simulink model "building_HVAC_V00_027_AI_2019b"  (R2021b)
settings: Solver=ode3  StartTime=1425600  StopTime=1429297  FixedStep=0.1  RelTol=1e-3
model workspace (MAT data in the model file):
  A = 0
  pystep = 1
values from neighbouring files (symbols this model uses):
  Air_Cp = [1007 1007 1006 1006 1006 1006 1006 1006 1006 1006 1007 1007 ... (21 elements, 21x1)]    [data_07.mat]    (also in data_08.mat)
  Air_density = [1.783 1.582 1.422 1.367 1.341 1.316 1.292 1.268 1.246 1.225 1.204 1.184 ... (32 elements, 32x1)]    [data_07.mat]    (also in data_08.mat)
  Air_dynamic_viscosity_PaS = [1.318e-05 1.456e-05 1.588e-05 1.64e-05 1.665e-05 1.69e-05 1.715e-05 1.74e-05 1.764e-05 1.789e-05 1.813e-05 1.837e-05 ... (32 elements, 32x1)]    [data_07.mat]    (also in data_08.mat)
  Air_enthalpy = [325420 335490 345550 355620 365680 375730 385790 395850 405910 415970 426040 436110 ... (21 elements, 21x1)]    [data_07.mat]    (also in data_08.mat)
  Air_prandtl_number = [0.734 0.72 0.711 0.707 0.705 0.701 0.699 0.698 0.699 0.702]    [data_07.mat]    (also in data_08.mat)
  Air_Temp_for_Cp = [200 210 220 230 240 250 260 270 280 290 300 310 ... (21 elements, 21x1)]    [data_07.mat]    (also in data_08.mat)
  Air_Temp_for_density = [-75 -50 -25 -15 -10 -5 0 5 10 15 20 25 ... (32 elements, 32x1)]    [data_07.mat]    (also in data_08.mat)
  Air_Temp_for_dynamic_viscosity = [-75 -50 -25 -15 -10 -5 0 5 10 15 20 25 ... (32 elements, 32x1)]    [data_07.mat]    (also in data_08.mat)
  Air_Temp_for_enthalpy = [200 210 220 230 240 250 260 270 280 290 300 310 ... (21 elements, 21x1)]    [data_07.mat]    (also in data_08.mat)
  Air_Temp_for_prandtl_number = [-100 -50 0 25 50 100 150 200 250 300]    [data_07.mat]    (also in data_08.mat)
  Air_Temp_for_thermal_conductivity = [-190 -150 -100 -75 -50 -25 -15 -10 -5 0 5 10 ... (35 elements, 35x1)]    [data_07.mat]    (also in data_08.mat)
  Air_thermal_conductivity = [0.00782 0.01169 0.0162 0.01834 0.02041 0.02241 0.0232 0.02359 0.02397 0.02436 0.02474 0.02512 ... (35 elements, 35x1)]    [data_07.mat]    (also in data_08.mat)
  Ambient_Solar_heat_Seoul_20200701_to_20200731 = [0 0 0 0 0 0 2.777777778 38.88888889 72.22222222 97.22222222 333.3333333 263.8888889 ... (745 elements, 745x1)]    [data_07.mat]    (also in data_08.mat)
  Ambient_Solar_heat_Seoul_20200701_to_20210630 = [0 0 0 0 0 2.777777778 38.88888889 72.22222222 97.22222222 333.3333333 263.8888889 152.7777778 ... (8736 elements, 8736x1)]    [data_07.mat]    (also in data_08.mat)
  Ambient_Solar_heat_Seoul_20200801_to_20200831 = [0 0 0 0 0 0 2.777777778 11.11111111 38.88888889 63.88888889 127.7777778 258.3333333 ... (745 elements, 745x1)]    [data_07.mat]    (also in data_08.mat)
  Ambient_Solar_heat_Seoul_20200901_to_20200930 = [0 0 0 0 0 0 0 22.22222222 108.3333333 141.6666667 211.1111111 386.1111111 ... (721 elements, 721x1)]    [data_07.mat]    (also in data_08.mat)
  Ambient_Temp_Seoul_20200701_to_20200731 = [18.8 18.8 18.7 18.4 18.2 18.2 18.3 18.5 19.1 19.6 21.2 21.6 ... (745 elements, 745x1)]    [data_07.mat]    (also in data_08.mat)
  Ambient_Temp_Seoul_20200701_to_20210630 = [18.8 18.7 18.4 18.2 18.2 18.3 18.5 19.1 19.6 21.2 21.6 21.7 ... (8736 elements, 8736x1)]    [data_07.mat]    (also in data_08.mat)
  Ambient_Temp_Seoul_20200801_to_20200831 = [25 24.6 24.6 24.7 24.7 24.5 24.3 24.3 24.6 25 25.7 26.8 ... (745 elements, 745x1)]    [data_07.mat]    (also in data_08.mat)
  Ambient_Temp_Seoul_20200901_to_20200930 = [26.2 25.8 25.5 24.9 24.5 24.3 24 23.9 24.4 24.8 25.7 26.6 ... (721 elements, 721x1)]    [data_07.mat]    (also in data_08.mat)
  Ambient_Time_Seoul_20200701_to_20200731 = [0 3600 7200 10800 14400 18000 21600 25200 28800 32400 36000 39600 ... (745 elements, 745x1)]    [data_07.mat]    (also in data_08.mat)
  Ambient_Time_Seoul_20200701_to_20210630 = [0 3600 7200 10800 14400 18000 21600 25200 28800 32400 36000 39600 ... (8736 elements, 8736x1)]    [data_07.mat]    (also in data_08.mat)
  Ambient_Time_Seoul_20200901_to_20200930 = [0 3600 7200 10800 14400 18000 21600 25200 28800 32400 36000 39600 ... (721 elements, 721x1)]    [data_07.mat]    (also in data_08.mat)
  Ambient_Water_Vapor_Pressure_Seoul_20200701_to_20200731 = [18.4 18.8 18.6 18.2 17.9 17.7 18.6 18.6 18.5 19.1 19.9 19.5 ... (745 elements, 745x1)]    [data_07.mat]    (also in data_08.mat)
  Ambient_Water_Vapor_Pressure_Seoul_20200701_to_20210630 = [18.8 18.6 18.2 17.9 17.7 18.6 18.6 18.5 19.1 19.9 19.5 19.4 ... (8736 elements, 8736x1)]    [data_07.mat]    (also in data_08.mat)
  Ambient_Water_Vapor_Pressure_Seoul_20200801_to_20200831 = [28.4 27.7 28.1 28.8 29.1 28.8 28.8 29.1 29.7 30 31.3 29.8 ... (745 elements, 745x1)]    [data_07.mat]    (also in data_08.mat)
  Ambient_Water_Vapor_Pressure_Seoul_20200901_to_20200930 = [26.1 25.8 25.6 24.7 24 24.3 22.9 23.1 23.1 22.8 24 24.3 ... (721 elements, 721x1)]    [data_07.mat]    (also in data_08.mat)
  Ambient_wind_speed_Seoul_20200701_to_20200731 = [3.7 3 3 2.3 1.2 1.5 3.1 1.4 1 1.4 2.5 2.1 ... (745 elements, 745x1)]    [data_07.mat]    (also in data_08.mat)
  Ambient_wind_speed_Seoul_20200701_to_20210630 = [3 3 2.3 1.2 1.5 3.1 1.4 1 1.4 2.5 2.1 2 ... (8736 elements, 8736x1)]    [data_07.mat]    (also in data_08.mat)
  Ambient_wind_speed_Seoul_20200801_to_20200831 = [3.4 0.5 0.5 1.2 0.8 1.3 1.8 1.4 1.2 1.1 1.8 3.4 ... (745 elements, 745x1)]    [data_07.mat]    (also in data_08.mat)
  Ambient_wind_speed_Seoul_20200901_to_20200930 = [2.3 2.2 2.5 2.6 2.4 2.1 1.7 2.7 2.6 2.5 1.5 1.8 ... (721 elements, 721x1)]    [data_07.mat]    (also in data_08.mat)
  init_time = start_time +60    [SIMULINK_RUn.m]    (also in data_07.mat = 0; data_08.mat = 1425660)
  Initial_Temp = 273 + 28    (= 301)    [SIMULINK_RUn.m]    (also in data_07.mat = 285; data_08.mat = 302)
  Shadow_20200701_to_20210630 = [285 300 315 330 345 360 15 30 45 60 75 90 ... (8736 elements, 8736x1)]    [data_07.mat]    (also in data_08.mat)
  start_time = 12 * 3600 + da * day_to_sec    [SIMULINK_RUn.m]    (also in data_07.mat = 0; data_08.mat = 1425600)
  Under_30cm_ground_Temp_Seoul_20200701_to_20200731 = [22.6 22.6 22.5 22.5 22.4 22.3 22.3 22.2 22.1 22.1 22 22 ... (745 elements, 745x1)]    [data_07.mat]    (also in data_08.mat)
  Under_30cm_ground_Temp_Seoul_20200701_to_20210630 = [22.6 22.5 22.5 22.4 22.3 22.3 22.2 22.1 22.1 22 22 22 ... (8736 elements, 8736x1)]    [data_07.mat]    (also in data_08.mat)
  Under_30cm_ground_Temp_Seoul_20200801_to_20200831 = [25.6 25.6 25.6 25.5 25.5 25.5 25.4 25.4 25.3 25.3 25.3 25.2 ... (745 elements, 745x1)]    [data_07.mat]    (also in data_08.mat)
  Under_30cm_ground_Temp_Seoul_20200901_to_20200930 = [27.4 27.4 27.4 27.4 27.3 27.3 27.3 27.2 27.2 27.1 27 27 ... (721 elements, 721x1)]    [data_07.mat]    (also in data_08.mat)
  water_saturation_enthalpy_latent = [2500899.39 2498955.8 2496540.3 2494128 2491818 2489411 2487006 2484604 2482303 2479905 2477508 2475213 ... (64 elements, 64x1)]    [data_07.mat]    (also in data_08.mat)
  water_saturation_enthalpy_vapor = [2500900 2502500 2504300 2506100 2508000 2509800 2511600 2513400 2515300 2517100 2518900 2520800 ... (64 elements, 64x1)]    [data_07.mat]    (also in data_08.mat)
  water_saturation_pressure = [611.65 650.03 698.46 750.07 805.02 863.5 925.7 991.83 1062.2 1136.8 1216 1300 ... (64 elements, 64x1)]    [data_07.mat]    (also in data_08.mat)
  water_Temp_for_saturation_enthalpy_latent = [273.16 274 275 276 277 278 279 280 281 282 283 284 ... (64 elements, 64x1)]    [data_07.mat]    (also in data_08.mat)
  water_Temp_for_saturation_enthalpy_vapor = [273.16 274 275 276 277 278 279 280 281 282 283 284 ... (64 elements, 64x1)]    [data_07.mat]    (also in data_08.mat)
  water_Temp_for_saturation_pressure = [273.16 274 275 276 277 278 279 280 281 282 283 284 ... (64 elements, 64x1)]    [data_07.mat]    (also in data_08.mat)
undefined symbols (not defined in the file or in its folder): DiscIntNeverNeededParam
libraries: fuzblock x1
(part 2 of 3)

== system building_HVAC_V00_027_AI_2019b/Building_Block/Blower_and_InnerAir_Block ==
  Infiltration_[m3/s] : Inport
  Ventilation_[m3/s] : Inport  Port=2
  Ambient_temperature_[K]1 : Inport  Port=3
  Ambient_water_vapor_pressure_[Pa] : Inport  Port=4
  Blower_volume_flow_rate_[m3/s] : Inport  Port=5
  Q_AC_cooling_[W] : Inport  Port=6
  AC_ON : Inport  Port=7
  AC_Condensation_Mass_Flow_Rate_[kg/s]_Block : Subsystem
  AC_Outlet_Q_[W]_Block : Subsystem
  Absolute_Humidity_[-]_Block : Subsystem
  Air_Mass_Flow_Rate Infiltration InnerAir : Subsystem
  Air_Mass_Flow_Rate Ventilation InnerAir : Subsystem
  Blower_Mass_Flow_Rate_[kg/s] Water_and_Air : Subsystem
  Blower_Q_[W]_Block : Subsystem
  InnerAir_DewPoint_Temperature_[K]_Block : Subsystem
  InnerAir_H2O_Pressure_[Pa]_Block : Subsystem
  InnerAir_Temperature_Block : Subsystem
  Mass_H2O_vapor_InnerAir : Subsystem
  Mass_dry_air_InnerAir : Subsystem
  Water_Mass_Flow_Rate Infiltration InnerAir : Subsystem
  Water_Mass_Flow_Rate Ventilation InnerAir : Subsystem
  atmosperic pressure [Pa] : Constant  Value=101325
  gas constant dry air [J/kgK] : Constant  Value=287.05
  gas constant water [J/kgK] : Constant  Value=462.52
  InnerAir_temperature_[K] : Outport
  InnerAir_temperature_[degC] : Outport  Port=2
  tag scope: atmosphere_pressure=global, gas_constant_dry_air=global, gas_constant_water=global
  wires:
  atmosperic pressure [Pa]/1 -> [atmosphere_pressure]
  gas constant dry air [J/kgK]/1 -> [gas_constant_dry_air]
  gas constant water [J/kgK]/1 -> [gas_constant_water]
  Ventilation_[m3/s]/1 -> Water_Mass_Flow_Rate Ventilation InnerAir/1(Ventilation_[m3/s]), Air_Mass_Flow_Rate Ventilation InnerAir/1(Ventilation_[m3/s])
  Infiltration_[m3/s]/1 -> Water_Mass_Flow_Rate Infiltration InnerAir/3(Infiltration_[m3/s]), Air_Mass_Flow_Rate Infiltration InnerAir/1(Infiltration_[m3/s])
  Ambient_water_vapor_pressure_[Pa]/1 -> Water_Mass_Flow_Rate Infiltration InnerAir/1(Ambient_water_vapor_pressure_[Pa])
  Ambient_temperature_[K]1/1 -> Water_Mass_Flow_Rate Infiltration InnerAir/2(Ambient_temperature_[K]), Air_Mass_Flow_Rate Infiltration InnerAir/2(Ambient_temperature_[K]), Mass_H2O_vapor_InnerAir/1(Ambient_temperature_[K]2), Mass_dry_air_InnerAir/1(Ambient_temperature_[K]2)
  InnerAir_Temperature_Block/2(InnerAir_temperature_[degC]) -> InnerAir_temperature_[degC]/1
  Q_AC_cooling_[W]/1 -> AC_Condensation_Mass_Flow_Rate_[kg/s]_Block/1(Q_AC_cooling_[W])
  AC_ON/1 -> AC_Condensation_Mass_Flow_Rate_[kg/s]_Block/2(AC_ON)
  Blower_volume_flow_rate_[m3/s]/1 -> Blower_Mass_Flow_Rate_[kg/s] Water_and_Air/2(Blower_volume_flow_rate_[m3/s])
  InnerAir_Temperature_Block/1(InnerAir_temperature_[K]) -> InnerAir_temperature_[K]/1, Water_Mass_Flow_Rate Ventilation InnerAir/2(Inner_air_temperature_[K]), Air_Mass_Flow_Rate Ventilation InnerAir/2(InnerAir_temperature_[K]), Blower_Q_[W]_Block/1(Inner_air_temperature_[K]2), Blower_Mass_Flow_Rate_[kg/s] Water_and_Air/1(Inner_air_temperature_[K]1)

== system building_HVAC_V00_027_AI_2019b/Building_Block/East_Wall_Block ==
  Ambient_temperature_[K] : Inport
  Inner_air_temperature_[K] : Inport  Port=2
  Subsystem1 : Subsystem
  Subsystem2 : Subsystem
  Subsystem3 : Subsystem
  Subsystem4 : Subsystem
  East_outer_concrete_wall_temperature_[degC] : Outport
  East_insulator_temperature_[degC] : Outport  Port=2
  East_inner_concrete_wall_temperature_[degC] : Outport  Port=3
  Q_East_InnerWall_to_InnerAir_[W] : Outport  Port=4
  wires:
  Subsystem3/2(East_inner_concrete_wall_temperature_[degC]) -> East_inner_concrete_wall_temperature_[degC]/1
  Inner_air_temperature_[K]/1 -> Subsystem1/2(Inner_air_temperature_[K]), Subsystem3/2(Inner_air_temperature_[K])
  Subsystem4/2(East_insulator_temperature_[degC]) -> East_insulator_temperature_[degC]/1
  Subsystem1/1(Q_East_InnerWall_to_InnerAir_[W]) -> Q_East_InnerWall_to_InnerAir_[W]/1
  [Inside] -> Subsystem3/3(East_Inner_Convective_coefficient_h), Subsystem1/3(East_Inner_Convective_coefficient_h)
  Subsystem2/1(East_outer_concrete_wall_temperature_[K]) -> Subsystem4/1(East_Outer_concrete_wall_temperature_[K])
  Subsystem4/1(East_insulator_temperature_[K]) -> Subsystem3/1(East_Insulator_temperature_[K]), Subsystem2/2(East_Insulator_temperature_[K])
  Ambient_temperature_[K]/1 -> Subsystem2/1(Ambient_temperature_[K])
  [Outside_East_West] -> Subsystem2/3(East_Out_Convective_coefficient_h)
  Subsystem2/2(East_outer_concrete_wall_temperature_[degC]) -> East_outer_concrete_wall_temperature_[degC]/1
  Subsystem3/1(East_inner_concrete_wall_temperature_[K]) -> Subsystem1/1(East_inner_concrete_wall_temperature_[K]), Subsystem4/2(East_Inner_concrete_wall_temperature_[K])

== system building_HVAC_V00_027_AI_2019b/Building_Block/Floorl_Block ==
  Under_30cm_soil_temperature_[K] : Inport
  Inner_air_temperature_[K] : Inport  Port=2
  Subsystem1 : Subsystem
  Subsystem3 : Subsystem
  Subsystem4 : Subsystem
  Floor_insulator_temperature_[degC] : Outport
  Floor_inner_wall_temperature_[degC] : Outport  Port=2
  Q_floor_to_InnerAir_[W] : Outport  Port=3
  wires:
  Subsystem3/1(Floor_inner_wall_temperature_[K]) -> Subsystem1/1(Floor_inner_concrete_wall_temperature_[K]), Subsystem4/2(Floor_Inner_concrete_wall_temperature_[K])
  Under_30cm_soil_temperature_[K]/1 -> Subsystem4/1(Under_30cm_soil_temperature_[K])
  Subsystem4/1(Floor_insulator_temperature_[K]) -> Subsystem3/1(Floor_Insulator_temperature_[K])
  [Inside] -> Subsystem1/3(West_Inner_Convective_coefficient_h), Subsystem3/3(Floor_Inner_Convective_coefficient_h)
  Subsystem1/1(Q_Floor_InnerWall_to_InnerAir_[W]) -> Q_floor_to_InnerAir_[W]/1
  Subsystem4/2(Floor_insulator_temperature_[degC]) -> Floor_insulator_temperature_[degC]/1
  Inner_air_temperature_[K]/1 -> Subsystem1/2(Inner_air_temperature_[K]), Subsystem3/2(Inner_air_temperature_[K])
  Subsystem3/2(Floor_inner_wall_temperature_[degC]) -> Floor_inner_wall_temperature_[degC]/1

== system building_HVAC_V00_027_AI_2019b/Building_Block/North_Wall_Block ==
  Ambient_temperature_[K] : Inport
  Inner_air_temperature_[K] : Inport  Port=2
  Subsystem1 : Subsystem
  Subsystem2 : Subsystem
  Subsystem3 : Subsystem
  Subsystem4 : Subsystem
  North_outer_concrete_wall_temperature_[degC] : Outport
  North_insulator_temperature_[degC] : Outport  Port=2
  North_inner_concrete_wall_temperature_[degC] : Outport  Port=3
  Q_North_InnerWall_to_InnerAir_[W] : Outport  Port=4
  wires:
  Subsystem3/2(North_inner_concrete_wall_temperature_[degC]) -> North_inner_concrete_wall_temperature_[degC]/1
  Inner_air_temperature_[K]/1 -> Subsystem1/2(Inner_air_temperature_[K]), Subsystem3/2(Inner_air_temperature_[K])
  Subsystem4/2(North_insulator_temperature_[degC]) -> North_insulator_temperature_[degC]/1
  Subsystem1/1(Q_North_InnerWall_to_InnerAir_[W]) -> Q_North_InnerWall_to_InnerAir_[W]/1
  [Inside] -> Subsystem3/3(North_Inner_Convective_coefficient_h), Subsystem1/3(North_Inner_Convective_coefficient_h)
  Subsystem2/1(North_outer_concrete_wall_temperature_[K]) -> Subsystem4/1(North_Outer_concrete_wall_temperature_[K])
  Subsystem4/1(North_insulator_temperature_[K]) -> Subsystem3/1(North_Insulator_temperature_[K]), Subsystem2/2(North_Insulator_temperature_[K])
  Ambient_temperature_[K]/1 -> Subsystem2/1(Ambient_temperature_[K])
  [Outside_South_North] -> Subsystem2/3(North_Out_Convective_coefficient_h)
  Subsystem2/2(North_outer_concrete_wall_temperature_[degC]) -> North_outer_concrete_wall_temperature_[degC]/1
  Subsystem3/1(North_inner_concrete_wall_temperature_[K]) -> Subsystem1/1(North_inner_concrete_wall_temperature_[K]), Subsystem4/2(North_Inner_concrete_wall_temperature_[K])

== system building_HVAC_V00_027_AI_2019b/Building_Block/South_Wall_Block ==
  Ambient_temperature_[K] : Inport
  Inner_air_temperature_[K] : Inport  Port=2
  Subsystem1 : Subsystem
  Subsystem2 : Subsystem
  Subsystem3 : Subsystem
  Subsystem4 : Subsystem
  South_outer_concrete_wall_temperature_[degC] : Outport
  South_insulator_temperature_[degC] : Outport  Port=2
  South_inner_concrete_wall_temperature_[degC] : Outport  Port=3
  Q_South_InnerWall_to_InnerAir_[W] : Outport  Port=4
  wires:
  Subsystem3/1(South_inner_concrete_wall_temperature_[K]) -> Subsystem1/1(South_inner_concrete_wall_temperature_[K]), Subsystem4/2(South_Inner_concrete_wall_temperature_[K])
  Subsystem2/2(South_outer_concrete_wall_temperature_[degC]) -> South_outer_concrete_wall_temperature_[degC]/1
  [Outside_South_North] -> Subsystem2/3(South_Out_Convective_coefficient_h)
  Ambient_temperature_[K]/1 -> Subsystem2/1(Ambient_temperature_[K])
  Subsystem4/1(South_insulator_temperature_[K]) -> Subsystem2/2(South_Insulator_temperature_[K]), Subsystem3/1(South_Insulator_temperature_[K])
  Subsystem2/1(South_outer_concrete_wall_temperature_[K]) -> Subsystem4/1(South_Outer_concrete_wall_temperature_[K])
  [Inside] -> Subsystem3/3(South_Inner_Convective_coefficient_h), Subsystem1/3(South_Inner_Convective_coefficient_h)
  Subsystem1/1(Q_South_InnerWall_to_InnerAir_[W]) -> Q_South_InnerWall_to_InnerAir_[W]/1
  Subsystem4/2(South_insulator_temperature_[degC]) -> South_insulator_temperature_[degC]/1
  Inner_air_temperature_[K]/1 -> Subsystem3/2(Inner_air_temperature_[K]), Subsystem1/2(Inner_air_temperature_[K])
  Subsystem3/2(South_inner_concrete_wall_temperature_[degC]) -> South_inner_concrete_wall_temperature_[degC]/1

== system building_HVAC_V00_027_AI_2019b/Building_Block/Subsystem ==
  Density : Inport
  Wind speed (m/s) : Inport  Port=2
  Dynamic viscosity : Inport  Port=3
  Ptandtl number : Inport  Port=4
  Air Thermal conductivity(W/mK) : Inport  Port=5
  Characteristic_length_(m) L : Inport  Port=6
  "Convective_coefficient_(W/(m2)K) h=(Nu)x(k)/(L) Frank P. Incropera and David P. DeWitt, \"Fundamentals of Heat and Mass Transfer\", (1996), FOURTH EDITION, pg. 320" : Fcn  Expr=u(1)/u(2)*u(3)
  Mux1 : Mux
  Mux2 : Mux  Inputs=2
  Mux3 : Mux  Inputs=3
  "Nusselt_number_(-) Nu [laminar_flow] Frank P. Incropera and David P. DeWitt, \"Fundamentals of Heat and Mass Transfer\", (1996), FOURTH EDITION, pg. 354" : Fcn  Expr=0.664*(u(1)^(1/2))*(u(2)^(1/3))
  "Nusselt_number_(-) Nu [turbulent_flow] Frank P. Incropera and David P. DeWitt, \"Fundamentals of Heat and Mass Transfer\", (1996), FOURTH EDITION, pg. 355" : Fcn  Expr=0.0296*(u(1)^(4/5))*(u(2)^(1/3))
  Reynold_number_(-) Re : Fcn  Expr=u(1)*u(2)*u(3)/u(4)
  Switch1 : Switch  Criteria=u2 > Threshold  Threshold=10^8
  h (W/(m2)K) : Outport  VectorParamsAs1DForOutWhenUnconnected=off
  wires:
  Mux2/1 -> "Nusselt_number_(-) Nu [turbulent_flow] Frank P. Incropera and David P. DeWitt, \"Fundamentals of Heat and Mass Transfer\", (1996), FOURTH EDITION, pg. 355"/1, "Nusselt_number_(-) Nu [laminar_flow] Frank P. Incropera and David P. DeWitt, \"Fundamentals of Heat and Mass Transfer\", (1996), FOURTH EDITION, pg. 354"/1
  "Nusselt_number_(-) Nu [laminar_flow] Frank P. Incropera and David P. DeWitt, \"Fundamentals of Heat and Mass Transfer\", (1996), FOURTH EDITION, pg. 354"/1 -> Switch1/3
  "Nusselt_number_(-) Nu [turbulent_flow] Frank P. Incropera and David P. DeWitt, \"Fundamentals of Heat and Mass Transfer\", (1996), FOURTH EDITION, pg. 355"/1 -> Switch1/1
  Mux1/1 -> Reynold_number_(-) Re/1
  Characteristic_length_(m) L/1 -> Mux3/2, Mux1/3
  Mux3/1 -> "Convective_coefficient_(W/(m2)K) h=(Nu)x(k)/(L) Frank P. Incropera and David P. DeWitt, \"Fundamentals of Heat and Mass Transfer\", (1996), FOURTH EDITION, pg. 320"/1
  Ptandtl number/1 -> Mux2/2
  Switch1/1 -> Mux3/1
  Reynold_number_(-) Re/1 -> Switch1/2, Mux2/1
  Dynamic viscosity/1 -> Mux1/4
  Air Thermal conductivity(W/mK)/1 -> Mux3/3
  Density/1 -> Mux1/1
  "Convective_coefficient_(W/(m2)K) h=(Nu)x(k)/(L) Frank P. Incropera and David P. DeWitt, \"Fundamentals of Heat and Mass Transfer\", (1996), FOURTH EDITION, pg. 320"/1 -> h (W/(m2)K)/1
  Wind speed (m/s)/1 -> Mux1/2

== system building_HVAC_V00_027_AI_2019b/Building_Block/Subsystem1 ==
  Density : Inport
  Wind speed (m/s) : Inport  Port=2
  Dynamic viscosity : Inport  Port=3
  Ptandtl number : Inport  Port=4
  Air Thermal conductivity(W/mK) : Inport  Port=5
  Characteristic_length_(m) L : Inport  Port=6
  "Convective_coefficient_(W/(m2)K) h=(Nu)x(k)/(L) Frank P. Incropera and David P. DeWitt, \"Fundamentals of Heat and Mass Transfer\", (1996), FOURTH EDITION, pg. 320" : Fcn  Expr=u(1)/u(2)*u(3)
  Mux1 : Mux
  Mux2 : Mux  Inputs=2
  Mux3 : Mux  Inputs=3
  "Nusselt_number_(-) Nu [laminar_flow] Frank P. Incropera and David P. DeWitt, \"Fundamentals of Heat and Mass Transfer\", (1996), FOURTH EDITION, pg. 354" : Fcn  Expr=0.664*(u(1)^(1/2))*(u(2)^(1/3))
  "Nusselt_number_(-) Nu [turbulent_flow] Frank P. Incropera and David P. DeWitt, \"Fundamentals of Heat and Mass Transfer\", (1996), FOURTH EDITION, pg. 355" : Fcn  Expr=0.0296*(u(1)^(4/5))*(u(2)^(1/3))
  Reynold_number_(-) Re : Fcn  Expr=u(1)*u(2)*u(3)/u(4)
  Switch1 : Switch  Criteria=u2 > Threshold  Threshold=10^8
  h (W/(m2)K) : Outport  VectorParamsAs1DForOutWhenUnconnected=off
  wires:
  Wind speed (m/s)/1 -> Mux1/2
  "Convective_coefficient_(W/(m2)K) h=(Nu)x(k)/(L) Frank P. Incropera and David P. DeWitt, \"Fundamentals of Heat and Mass Transfer\", (1996), FOURTH EDITION, pg. 320"/1 -> h (W/(m2)K)/1
  Density/1 -> Mux1/1
  Air Thermal conductivity(W/mK)/1 -> Mux3/3
  Dynamic viscosity/1 -> Mux1/4
  Reynold_number_(-) Re/1 -> Mux2/1, Switch1/2
  Switch1/1 -> Mux3/1
  Ptandtl number/1 -> Mux2/2
  Mux3/1 -> "Convective_coefficient_(W/(m2)K) h=(Nu)x(k)/(L) Frank P. Incropera and David P. DeWitt, \"Fundamentals of Heat and Mass Transfer\", (1996), FOURTH EDITION, pg. 320"/1
  Characteristic_length_(m) L/1 -> Mux1/3, Mux3/2
  Mux1/1 -> Reynold_number_(-) Re/1
  "Nusselt_number_(-) Nu [turbulent_flow] Frank P. Incropera and David P. DeWitt, \"Fundamentals of Heat and Mass Transfer\", (1996), FOURTH EDITION, pg. 355"/1 -> Switch1/1
  "Nusselt_number_(-) Nu [laminar_flow] Frank P. Incropera and David P. DeWitt, \"Fundamentals of Heat and Mass Transfer\", (1996), FOURTH EDITION, pg. 354"/1 -> Switch1/3
  Mux2/1 -> "Nusselt_number_(-) Nu [laminar_flow] Frank P. Incropera and David P. DeWitt, \"Fundamentals of Heat and Mass Transfer\", (1996), FOURTH EDITION, pg. 354"/1, "Nusselt_number_(-) Nu [turbulent_flow] Frank P. Incropera and David P. DeWitt, \"Fundamentals of Heat and Mass Transfer\", (1996), FOURTH EDITION, pg. 355"/1

== system building_HVAC_V00_027_AI_2019b/Building_Block/West_Wall_Block ==
  Ambient_temperature_[K] : Inport
  Inner_air_temperature_[K] : Inport  Port=2
  Subsystem1 : Subsystem
  Subsystem2 : Subsystem
  Subsystem3 : Subsystem
  Subsystem4 : Subsystem
  West_outer_concrete_wall_temperature_[degC] : Outport
  West_insulator_temperature_[degC] : Outport  Port=2
  West_inner_concrete_wall_temperature_[degC] : Outport  Port=3
  Q_West_InnerWall_to_InnerAir_[W] : Outport  Port=4
  wires:
  Subsystem3/1(West_inner_concrete_wall_temperature_[K]) -> Subsystem1/1(West_inner_concrete_wall_temperature_[K]), Subsystem4/2(West_Inner_concrete_wall_temperature_[K])
  Subsystem2/2(West_outer_concrete_wall_temperature_[degC]) -> West_outer_concrete_wall_temperature_[degC]/1
  [Outside_East_West] -> Subsystem2/3(West_Out_Convective_coefficient_h)
  Ambient_temperature_[K]/1 -> Subsystem2/1(Ambient_temperature_[K])
  Subsystem4/1(West_insulator_temperature_[K]) -> Subsystem2/2(West_Insulator_temperature_[K]), Subsystem3/1(West_Insulator_temperature_[K])
  Subsystem2/1(West_outer_concrete_wall_temperature_[K]) -> Subsystem4/1(West_Outer_concrete_wall_temperature_[K])
  [Inside] -> Subsystem1/3(West_Inner_Convective_coefficient_h), Subsystem3/3(West_Inner_Convective_coefficient_h)
  Subsystem1/1(Q_West_InnerWall_to_InnerAir_[W]) -> Q_West_InnerWall_to_InnerAir_[W]/1
  Subsystem4/2(West_insulator_temperature_[degC]) -> West_insulator_temperature_[degC]/1
  Inner_air_temperature_[K]/1 -> Subsystem1/2(Inner_air_temperature_[K]), Subsystem3/2(Inner_air_temperature_[K])
  Subsystem3/2(West_inner_concrete_wall_temperature_[degC]) -> West_inner_concrete_wall_temperature_[degC]/1

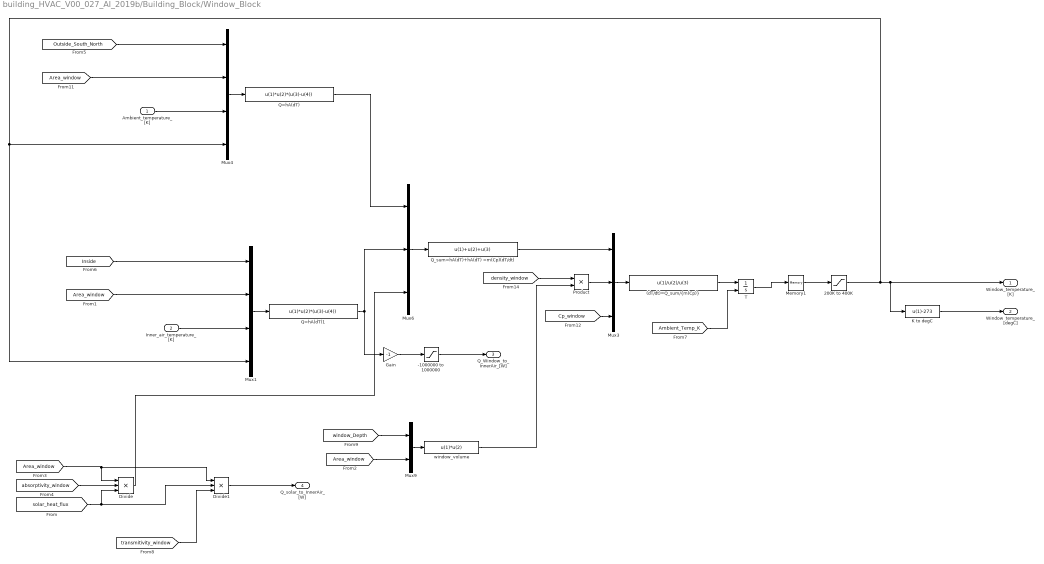
== system building_HVAC_V00_027_AI_2019b/Building_Block/Window_Block ==
  Ambient_temperature_[K] : Inport
  Inner_air_temperature_[K] : Inport  Port=2
  "(dT/dt)=Q_sum/{m(Cp)}" : Fcn  Expr=u(1)/u(2)/u(3)
  -1000000 to 1000000 : Saturate  UpperLimit=1000000  LowerLimit=-1000000
  200K to 400K : Saturate  UpperLimit=400  LowerLimit=200
  Divide : Product  Inputs=***
  Divide1 : Product  Inputs=***
  Gain : Gain  Gain=-1
  K to degC : Fcn  Expr=u(1)-273
  Memory1 : Memory  InitialCondition=300  InheritSampleTime=on
  Mux1 : Mux
  Mux3 : Mux  Inputs=3
  Mux4 : Mux
  Mux6 : Mux  Inputs=3
  Mux9 : Mux  Inputs=2
  Product : Product
  Q=hA(dT) : Fcn  Expr=u(1)*u(2)*(u(3)-u(4))
  Q=hA(dT)1 : Fcn  Expr=u(1)*u(2)*(u(3)-u(4))
  Q_sum=hA(dT)+hA(dT) =m(Cp)(dT/dt) : Fcn  Expr=u(1)+u(2)+u(3)
  T : Integrator  InitialConditionSource=external
  window_volume : Fcn  Expr=u(1)*u(2)
  Window_temperature_[K] : Outport
  Window_temperature_[degC] : Outport  Port=2
  Q_Window_to_InnerAir_[W] : Outport  Port=3
  Q_solar_to_InnerAir_[W] : Outport  Port=4
  wires:
  Mux6/1 -> Q_sum=hA(dT)+hA(dT) =m(Cp)(dT/dt)/1
  Mux3/1 -> "(dT/dt)=Q_sum/{m(Cp)}"/1
  [density_window] -> Product/1
  Mux9/1 -> window_volume/1
  "(dT/dt)=Q_sum/{m(Cp)}"/1 -> T/1
  [Cp_window] -> Mux3/3
  Product/1 -> Mux3/2
  [window_Depth] -> Mux9/1
  [Area_window] -> Mux9/2
  T/1 -> Memory1/1
  Q=hA(dT)1/1 -> Gain/1, Mux6/2
  Memory1/1 -> 200K to 400K/1
  Q=hA(dT)/1 -> Mux6/1
  Q_sum=hA(dT)+hA(dT) =m(Cp)(dT/dt)/1 -> Mux3/1
  window_volume/1 -> Product/2
  K to degC/1 -> Window_temperature_[degC]/1
  [Area_window] -> Mux4/2
  Ambient_temperature_[K]/1 -> Mux4/3
  Mux4/1 -> Q=hA(dT)/1
  [Outside_South_North] -> Mux4/1
  200K to 400K/1 -> Mux4/4, Mux1/4, K to degC/1, Window_temperature_[K]/1
  [Inside] -> Mux1/1
  Mux1/1 -> Q=hA(dT)1/1
  Inner_air_temperature_[K]/1 -> Mux1/3
  [Area_window] -> Mux1/2
  -1000000 to 1000000/1 -> Q_Window_to_InnerAir_[W]/1
  Gain/1 -> -1000000 to 1000000/1
  Divide/1 -> Mux6/3
  Divide1/1 -> Q_solar_to_InnerAir_[W]/1
  [Area_window] -> Divide1/1, Divide/1
  [solar_heat_flux] -> Divide1/2, Divide/3
  [absorptivity_window] -> Divide/2
  [Ambient_Temp_K] -> T/2
  [transmitivity_window] -> Divide1/3

== system building_HVAC_V00_027_AI_2019b/Building_Block/Blower_and_InnerAir_Block/AC_Condensation_Mass_Flow_Rate_[kg//s]_Block ==
  Q_AC_cooling_[W] : Inport
  AC_ON : Inport  Port=2
  Divide : Product  Inputs=**/
  Latent_enthalpy_of_saturated_water_(J/kg) of temperature_(K)1 : Lookup_n-D  NumberOfTableDimensions=1  BreakpointsForDimension1=water_Temp_for_saturation_enthalpy_latent  Table=water_saturation_enthalpy_latent  InternalRulePriority=Speed  RndMeth=Simplest  InputSameDT=on
  Saturation1 : Saturate  UpperLimit=100  LowerLimit=0
  Saturation5 : Saturate  UpperLimit=400  LowerLimit=273.16
  Scope25 : Scope
  "[J/kg]" : Gain
  "[K]1" : Gain
  "[W]" : Gain
  "[kg/s]1" : Gain
  tag scope: AC_condensation_mass_flow=global
  wires:
  Divide/1 -> Saturation1/1
  [dewpoint_temperature_H2O_vapor] -> "[K]1"/1
  "[J/kg]"/1 -> Divide/3
  "[K]1"/1 -> Saturation5/1
  "[kg/s]1"/1 -> Scope25/1, [AC_condensation_mass_flow]
  Saturation5/1 -> Latent_enthalpy_of_saturated_water_(J/kg) of temperature_(K)1/1
  Latent_enthalpy_of_saturated_water_(J/kg) of temperature_(K)1/1 -> "[J/kg]"/1
  Q_AC_cooling_[W]/1 -> "[W]"/1
  AC_ON/1 -> Divide/1
  "[W]"/1 -> Divide/2
  Saturation1/1 -> "[kg/s]1"/1

== system building_HVAC_V00_027_AI_2019b/Building_Block/Blower_and_InnerAir_Block/AC_Outlet_Q_[W]_Block ==
  Add1 : Sum
  Add2 : Sum  Inputs=+-
  Divide2 : Product  Inputs=**
  Divide3 : Product  Inputs=**
  Enthalpy_of_air_(J/kg) of temperature_(K)1 : Lookup_n-D  NumberOfTableDimensions=1  BreakpointsForDimension1=Air_Temp_for_enthalpy  Table=Air_enthalpy  InternalRulePriority=Speed  RndMeth=Simplest  InputSameDT=on
  Enthalpy_of_saturated_water_vapor_(J/kg) of temperature_(K)1 : Lookup_n-D  NumberOfTableDimensions=1  BreakpointsForDimension1=water_Temp_for_saturation_enthalpy_vapor  Table=water_saturation_enthalpy_vapor  InternalRulePriority=Speed  RndMeth=Simplest  InputSameDT=on
  Saturation3 : Saturate  UpperLimit=400  LowerLimit=273.16
  Saturation6 : Saturate  UpperLimit=400  LowerLimit=200
  Scope1 : Scope
  Scope2 : Scope
  Scope3 : Scope
  "[J/kg]2" : Gain
  "[J/kg]3" : Gain
  "[K]3" : Gain
  "[K]4" : Gain
  "[kg/s]3" : Gain
  "[kg/s]4" : Gain
  tag scope: AC_outlet_Q=global
  wires:
  [dewpoint_temperature_H2O_vapor] -> Scope3/1, "[K]4"/1, "[K]3"/1
  [Blower_mass_flow_rate_air] -> "[kg/s]4"/1
  Add2/1 -> Scope2/1, "[kg/s]3"/1
  "[J/kg]3"/1 -> Divide3/2
  Enthalpy_of_air_(J/kg) of temperature_(K)1/1 -> "[J/kg]3"/1
  Saturation6/1 -> Enthalpy_of_air_(J/kg) of temperature_(K)1/1
  Divide2/1 -> Add1/1
  "[K]4"/1 -> Saturation6/1
  "[J/kg]2"/1 -> Divide2/2
  Divide3/1 -> Add1/2
  Add1/1 -> [AC_outlet_Q], Scope1/1
  Enthalpy_of_saturated_water_vapor_(J/kg) of temperature_(K)1/1 -> "[J/kg]2"/1
  Saturation3/1 -> Enthalpy_of_saturated_water_vapor_(J/kg) of temperature_(K)1/1
  "[kg/s]3"/1 -> Divide2/1
  "[K]3"/1 -> Saturation3/1
  "[kg/s]4"/1 -> Divide3/1
  [Blower_mass_flow_rate_water] -> Add2/1
  [AC_condensation_mass_flow] -> Add2/2

== system building_HVAC_V00_027_AI_2019b/Building_Block/Blower_and_InnerAir_Block/Absolute_Humidity_[-]_Block ==
  M_H2O_vapor / M_dry_air : Fcn  Expr=u(1)/u(2)
  Mux1 : Mux  Inputs=2
  Saturation1 : Saturate  UpperLimit=1  LowerLimit=0
  tag scope: absolute_humidity=global
  wires:
  Mux1/1 -> M_H2O_vapor / M_dry_air/1
  [M_dry_air] -> Mux1/2
  M_H2O_vapor / M_dry_air/1 -> Saturation1/1
  [M_H20_vapor] -> Mux1/1
  Saturation1/1 -> [absolute_humidity]

== system building_HVAC_V00_027_AI_2019b/Building_Block/Blower_and_InnerAir_Block/Air_Mass_Flow_Rate Infiltration InnerAir ==
  Infiltration_[m3/s] : Inport
  Ambient_temperature_[K] : Inport  Port=2
  Mux8 : Mux
  m_dot = P(V_dot)/R/T : Fcn  Expr=u(1)*u(2)/u(3)/u(4)
  tag scope: Infiltration_air=global
  wires:
  [atmosphere_pressure] -> Mux8/1
  [gas_constant_dry_air] -> Mux8/3
  Mux8/1 -> m_dot = P(V_dot)/R/T/1
  m_dot = P(V_dot)/R/T/1 -> [Infiltration_air]
  Ambient_temperature_[K]/1 -> Mux8/4
  Infiltration_[m3/s]/1 -> Mux8/2

== system building_HVAC_V00_027_AI_2019b/Building_Block/Blower_and_InnerAir_Block/Air_Mass_Flow_Rate Ventilation InnerAir ==
  Ventilation_[m3/s] : Inport
  InnerAir_temperature_[K] : Inport  Port=2
  Mux9 : Mux
  m_dot = P(V_dot)/R/T1 : Fcn  Expr=u(1)*u(2)/u(3)/u(4)
  tag scope: Ventilation_air=global
  wires:
  m_dot = P(V_dot)/R/T1/1 -> [Ventilation_air]
  [gas_constant_dry_air] -> Mux9/3
  [pressure_H2O_vapor] -> Mux9/1
  Mux9/1 -> m_dot = P(V_dot)/R/T1/1
  Ventilation_[m3/s]/1 -> Mux9/2
  InnerAir_temperature_[K]/1 -> Mux9/4

== system building_HVAC_V00_027_AI_2019b/Building_Block/Blower_and_InnerAir_Block/Blower_Mass_Flow_Rate_[kg//s] Water_and_Air ==
  Inner_air_temperature_[K]1 : Inport
  Blower_volume_flow_rate_[m3/s] : Inport  Port=2
  Mux12 : Mux
  Mux13 : Mux
  Scope1 : Scope
  Scope24 : Scope
  m_dot = P(V_dot)/R/T4 : Fcn  Expr=u(1)*u(2)/u(3)/u(4)
  m_dot = P(V_dot)/R/T5 : Fcn  Expr=u(1)*u(2)/u(3)/u(4)
  tag scope: Blower_mass_flow_rate_air=global, Blower_mass_flow_rate_water=global
  wires:
  [gas_constant_dry_air] -> Mux12/3
  Inner_air_temperature_[K]1/1 -> Mux12/4, Mux13/4
  [atmosphere_pressure] -> Mux12/1
  Blower_volume_flow_rate_[m3/s]/1 -> Mux13/2, Mux12/2
  Mux12/1 -> m_dot = P(V_dot)/R/T4/1
  Mux13/1 -> m_dot = P(V_dot)/R/T5/1
  [gas_constant_water] -> Mux13/3
  [pressure_H2O_vapor] -> Mux13/1
  m_dot = P(V_dot)/R/T4/1 -> Scope24/1, [Blower_mass_flow_rate_air]
  m_dot = P(V_dot)/R/T5/1 -> Scope1/1, [Blower_mass_flow_rate_water]

== system building_HVAC_V00_027_AI_2019b/Building_Block/Blower_and_InnerAir_Block/Blower_Q_[W]_Block ==
  Inner_air_temperature_[K]2 : Inport
  Add1 : Sum
  Divide2 : Product  Inputs=**
  Divide3 : Product  Inputs=**
  Enthalpy_of_air_(J/kg) of temperature_(K)2 : Lookup_n-D  NumberOfTableDimensions=1  BreakpointsForDimension1=Air_Temp_for_enthalpy  Table=Air_enthalpy  InternalRulePriority=Speed  RndMeth=Simplest  InputSameDT=on
  Enthalpy_of_saturated_water_vapor_(J/kg) of temperature_(K)1 : Lookup_n-D  NumberOfTableDimensions=1  BreakpointsForDimension1=water_Temp_for_saturation_enthalpy_vapor  Table=water_saturation_enthalpy_vapor  InternalRulePriority=Speed  RndMeth=Simplest  InputSameDT=on
  Saturation3 : Saturate  UpperLimit=400  LowerLimit=273.16
  Saturation6 : Saturate  UpperLimit=400  LowerLimit=200
  Scope24 : Scope
  "[J/kg]2" : Gain
  "[J/kg]3" : Gain
  "[K]3" : Gain
  "[K]4" : Gain
  "[kg/s]3" : Gain
  "[kg/s]4" : Gain
  tag scope: Blower_Q=global
  wires:
  Saturation3/1 -> Enthalpy_of_saturated_water_vapor_(J/kg) of temperature_(K)1/1
  [Blower_mass_flow_rate_water] -> "[kg/s]3"/1
  "[K]3"/1 -> Saturation3/1
  "[J/kg]2"/1 -> Divide2/2
  Inner_air_temperature_[K]2/1 -> "[K]4"/1, "[K]3"/1
  "[kg/s]4"/1 -> Divide3/1
  "[kg/s]3"/1 -> Divide2/1
  Add1/1 -> Scope24/1, [Blower_Q]
  [Blower_mass_flow_rate_air] -> "[kg/s]4"/1
  Divide3/1 -> Add1/2
  Enthalpy_of_saturated_water_vapor_(J/kg) of temperature_(K)1/1 -> "[J/kg]2"/1
  "[K]4"/1 -> Saturation6/1
  "[J/kg]3"/1 -> Divide3/2
  Enthalpy_of_air_(J/kg) of temperature_(K)2/1 -> "[J/kg]3"/1
  Saturation6/1 -> Enthalpy_of_air_(J/kg) of temperature_(K)2/1
  Divide2/1 -> Add1/1

== system building_HVAC_V00_027_AI_2019b/Building_Block/Blower_and_InnerAir_Block/InnerAir_DewPoint_Temperature_[K]_Block ==
  DewPoint_temperature_[K] of H2O_pressure_[Pa] : Lookup_n-D  NumberOfTableDimensions=1  BreakpointsForDimension1=water_saturation_pressure  Table=water_Temp_for_saturation_pressure  InternalRulePriority=Speed  RndMeth=Simplest  InputSameDT=on
  Saturation7 : Saturate  UpperLimit=245779  LowerLimit=611.65
  tag scope: dewpoint_temperature_H2O_vapor=global
  wires:
  Saturation7/1 -> DewPoint_temperature_[K] of H2O_pressure_[Pa]/1
  DewPoint_temperature_[K] of H2O_pressure_[Pa]/1 -> [dewpoint_temperature_H2O_vapor]
  [pressure_H2O_vapor] -> Saturation7/1

== system building_HVAC_V00_027_AI_2019b/Building_Block/Blower_and_InnerAir_Block/InnerAir_H2O_Pressure_[Pa]_Block ==
  Mux2 : Mux  Inputs=2
  "P_H2O_vapor = (omega)(P)/{0.622+omega}" : Fcn  Expr=u(1)*u(2)/(0.622+u(1))
  tag scope: pressure_H2O_vapor=global
  wires:
  [atmosphere_pressure] -> Mux2/2
  Mux2/1 -> "P_H2O_vapor = (omega)(P)/{0.622+omega}"/1
  "P_H2O_vapor = (omega)(P)/{0.622+omega}"/1 -> [pressure_H2O_vapor]
  [absolute_humidity] -> Mux2/1

== system building_HVAC_V00_027_AI_2019b/Building_Block/Blower_and_InnerAir_Block/InnerAir_Temperature_Block ==
  Air_Cp_(J/kgK) of temperature_(K) : Lookup_n-D  NumberOfTableDimensions=1  BreakpointsForDimension1=Air_Temp_for_Cp  Table=Air_Cp  InternalRulePriority=Speed  RndMeth=Simplest  InputSameDT=on
  Air_density_(kg/m3) of temperature_(degC) : Lookup_n-D  NumberOfTableDimensions=1  BreakpointsForDimension1=Air_Temp_for_density  Table=Air_density  InternalRulePriority=Speed  RndMeth=Simplest  InputSameDT=on
  Integrator : Integrator  InitialConditionSource=external
  Memory : Memory  InitialCondition=295  InheritSampleTime=on
  Mux5 : Mux  Inputs=3
  Mux6 : Mux  Inputs=2
  Saturation2 : Saturate  UpperLimit=400  LowerLimit=200
  Scope : Scope
  "[K] to [degC]" : Fcn  Expr=u(1)-273
  dT/dt = Q/m/(Cp) : Fcn  Expr=u(1)/u(2)/u(3)
  m = (rho)(V) : Fcn  Expr=u(1)*u(2)
  InnerAir_temperature_[K] : Outport
  InnerAir_temperature_[degC] : Outport  Port=2
  wires:
  m = (rho)(V)/1 -> Mux5/2
  [Volume_room] -> Mux6/2
  Integrator/1 -> Memory/1
  "[K] to [degC]"/1 -> InnerAir_temperature_[degC]/1, Air_density_(kg/m3) of temperature_(degC)/1
  Memory/1 -> Saturation2/1
  Saturation2/1 -> InnerAir_temperature_[K]/1, "[K] to [degC]"/1, Air_Cp_(J/kgK) of temperature_(K)/1
  Mux6/1 -> m = (rho)(V)/1
  [Q_total_to_InnerAir] -> Scope/1, Mux5/1
  Mux5/1 -> dT/dt = Q/m/(Cp)/1
  [Initial_inner_air_Temp] -> Integrator/2
  Air_density_(kg/m3) of temperature_(degC)/1 -> Mux6/1
  dT/dt = Q/m/(Cp)/1 -> Integrator/1
  Air_Cp_(J/kgK) of temperature_(K)/1 -> Mux5/3

== system building_HVAC_V00_027_AI_2019b/Building_Block/Blower_and_InnerAir_Block/Mass_H2O_vapor_InnerAir ==
  Ambient_temperature_[K]2 : Inport
  Integrator : Integrator  InitialConditionSource=external  InitialCondition=0.1
  Memory : Memory  InitialCondition=0.1
  Mux5 : Mux  Inputs=3
  Saturation : Saturate  UpperLimit=1000000  LowerLimit=0
  Scope25 : Scope
  Subsystem : Subsystem
  m_dot : Fcn  Expr=u(1)-u(2)-u(3)
  tag scope: M_H20_vapor=global
  wires:
  Saturation/1 -> Scope25/1, [M_H20_vapor]
  [Ventilation_water] -> Mux5/2
  m_dot/1 -> Integrator/1
  Integrator/1 -> Memory/1
  [AC_condensation_mass_flow] -> Mux5/3
  Memory/1 -> Saturation/1
  Mux5/1 -> m_dot/1
  [Infiltration_water] -> Mux5/1
  Subsystem/1(Out1) -> Integrator/2
  Ambient_temperature_[K]2/1 -> Subsystem/1(Ambient_temperature_[K]2)

== system building_HVAC_V00_027_AI_2019b/Building_Block/Blower_and_InnerAir_Block/Mass_dry_air_InnerAir ==
  Ambient_temperature_[K]2 : Inport
  Integrator1 : Integrator  InitialConditionSource=external  InitialCondition=0.1
  Memory1 : Memory  InitialCondition=0.1
  Mux6 : Mux  Inputs=2
  Saturation1 : Saturate  UpperLimit=1000000  LowerLimit=0
  Scope25 : Scope
  Subsystem1 : Subsystem
  m_dot1 : Fcn  Expr=u(1)-u(2)
  tag scope: M_dry_air=global
  wires:
  Integrator1/1 -> Memory1/1
  Subsystem1/1(Out1) -> Integrator1/2
  Saturation1/1 -> Scope25/1, [M_dry_air]
  [Ventilation_air] -> Mux6/2
  Memory1/1 -> Saturation1/1
  Mux6/1 -> m_dot1/1
  m_dot1/1 -> Integrator1/1
  [Infiltration_air] -> Mux6/1
  Ambient_temperature_[K]2/1 -> Subsystem1/1(Ambient_temperature_[K]2)

== system building_HVAC_V00_027_AI_2019b/Building_Block/Blower_and_InnerAir_Block/Water_Mass_Flow_Rate Infiltration InnerAir ==
  Ambient_water_vapor_pressure_[Pa] : Inport
  Ambient_temperature_[K] : Inport  Port=2
  Infiltration_[m3/s] : Inport  Port=3
  Mux10 : Mux
  m_dot = P(V_dot)/R/T2 : Fcn  Expr=u(1)*u(2)/u(3)/u(4)
  tag scope: Infiltration_water=global
  wires:
  Infiltration_[m3/s]/1 -> Mux10/2
  m_dot = P(V_dot)/R/T2/1 -> [Infiltration_water]
  [gas_constant_water] -> Mux10/3
  Mux10/1 -> m_dot = P(V_dot)/R/T2/1
  Ambient_water_vapor_pressure_[Pa]/1 -> Mux10/1
  Ambient_temperature_[K]/1 -> Mux10/4

== system building_HVAC_V00_027_AI_2019b/Building_Block/Blower_and_InnerAir_Block/Water_Mass_Flow_Rate Ventilation InnerAir ==
  Ventilation_[m3/s] : Inport
  Inner_air_temperature_[K] : Inport  Port=2
  Mux11 : Mux
  m_dot = P(V_dot)/R/T3 : Fcn  Expr=u(1)*u(2)/u(3)/u(4)
  tag scope: Ventilation_water=global
  wires:
  [atmosphere_pressure] -> Mux11/1
  [gas_constant_water] -> Mux11/3
  Ventilation_[m3/s]/1 -> Mux11/2
  m_dot = P(V_dot)/R/T3/1 -> [Ventilation_water]
  Mux11/1 -> m_dot = P(V_dot)/R/T3/1
  Inner_air_temperature_[K]/1 -> Mux11/4

== system building_HVAC_V00_027_AI_2019b/Building_Block/East_Wall_Block/Subsystem1 ==
  East_inner_concrete_wall_temperature_[K] : Inport
  Inner_air_temperature_[K] : Inport  Port=2
  East_Inner_Convective_coefficient_h : Inport  Port=3
  -1000000 to 1000000 : Saturate  UpperLimit=1000000  LowerLimit=-1000000
  Memory : Memory  InheritSampleTime=on
  Mux4 : Mux
  Q=hA(dT) : Fcn  Expr=u(1)*u(2)*(u(3)-u(4))
  Q_East_InnerWall_to_InnerAir_[W] : Outport
  wires:
  Memory/1 -> -1000000 to 1000000/1
  Q=hA(dT)/1 -> Memory/1
  Mux4/1 -> Q=hA(dT)/1
  -1000000 to 1000000/1 -> Q_East_InnerWall_to_InnerAir_[W]/1
  East_inner_concrete_wall_temperature_[K]/1 -> Mux4/3
  [Area_East] -> Mux4/2
  East_Inner_Convective_coefficient_h/1 -> Mux4/1
  Inner_air_temperature_[K]/1 -> Mux4/4

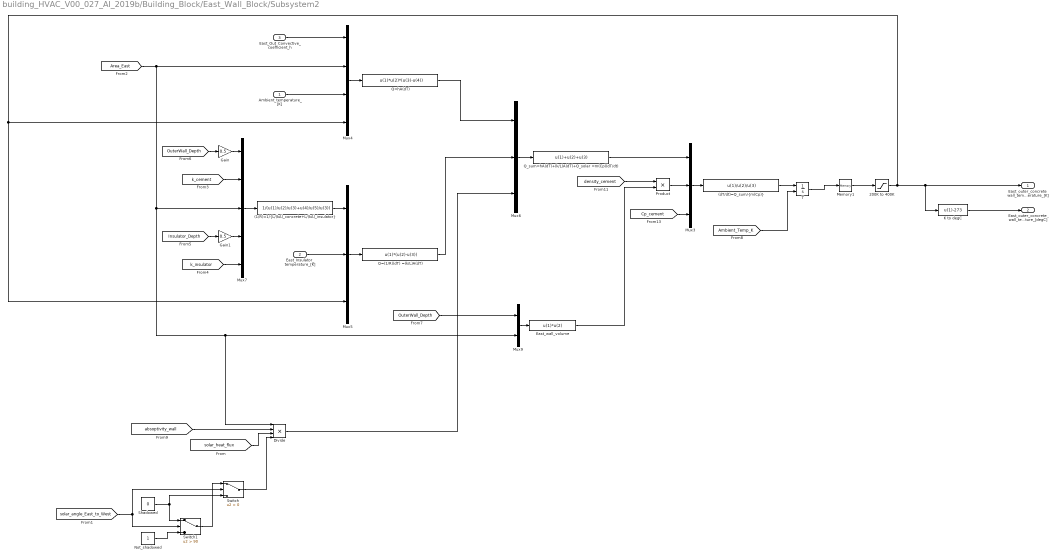
== system building_HVAC_V00_027_AI_2019b/Building_Block/East_Wall_Block/Subsystem2 ==
  Ambient_temperature_[K] : Inport
  East_Insulator_temperature_[K] : Inport  Port=2
  East_Out_Convective_coefficient_h : Inport  Port=3
  "(1/R)=1/{L/(kA)_concrete+L/(kA)_insulator}" : Fcn  Expr=1/(u(1)/u(2)/u(3)+u(4)/u(5)/u(3))
  "(dT/dt)=Q_sum/{m(Cp)}" : Fcn  Expr=u(1)/u(2)/u(3)
  200K to 400K : Saturate  UpperLimit=400  LowerLimit=200
  Divide : Product  Inputs=****
  East_wall_volume : Fcn  Expr=u(1)*u(2)
  Gain : Gain  Gain=0.5
  Gain1 : Gain  Gain=0.5
  K to degC : Fcn  Expr=u(1)-273
  Memory1 : Memory  InitialCondition=300  InheritSampleTime=on
  Mux3 : Mux  Inputs=3
  Mux4 : Mux
  Mux5 : Mux  Inputs=3
  Mux6 : Mux  Inputs=3
  Mux7 : Mux  Inputs=5
  Mux9 : Mux  Inputs=2
  Not_shadowed : Constant
  Product : Product
  Q=(1/R)(dT) =(k/L)A(dT) : Fcn  Expr=u(1)*(u(2)-u(3))
  Q=hA(dT) : Fcn  Expr=u(1)*u(2)*(u(3)-u(4))
  Q_sum=hA(dT)+(k/L)A(dT)+Q_solar =m(Cp)(dT/dt) : Fcn  Expr=u(1)+u(2)+u(3)
  Shadowed : Constant  Value=0
  Switch : Switch  Criteria=u2 > Threshold
  Switch1 : Switch  Criteria=u2 > Threshold  Threshold=90
  T : Integrator  InitialConditionSource=external
  East_outer_concrete_wall_temperature_[K] : Outport
  East_outer_concrete_wall_temperature_[degC] : Outport  Port=2
  wires:
  [absoptivity_wall] -> Divide/2
  [solar_heat_flux] -> Divide/3
  Divide/1 -> Mux6/3
  [Area_East] -> Mux4/2, Mux7/3, Divide/1, Mux9/2
  K to degC/1 -> East_outer_concrete_wall_temperature_[degC]/1
  East_wall_volume/1 -> Product/2
  [k_insulator] -> Mux7/5
  Gain1/1 -> Mux7/4
  East_Insulator_temperature_[K]/1 -> Mux5/2
  Q_sum=hA(dT)+(k/L)A(dT)+Q_solar =m(Cp)(dT/dt)/1 -> Mux3/1
  [k_cement] -> Mux7/2
  Mux7/1 -> "(1/R)=1/{L/(kA)_concrete+L/(kA)_insulator}"/1
  Q=hA(dT)/1 -> Mux6/1
  "(1/R)=1/{L/(kA)_concrete+L/(kA)_insulator}"/1 -> Mux5/1
  Gain/1 -> Mux7/1
  [Insulator_Depth] -> Gain1/1
  Memory1/1 -> 200K to 400K/1
  Q=(1/R)(dT) =(k/L)A(dT)/1 -> Mux6/2
  Mux4/1 -> Q=hA(dT)/1
  Mux5/1 -> Q=(1/R)(dT) =(k/L)A(dT)/1
  200K to 400K/1 -> Mux5/3, Mux4/4, East_outer_concrete_wall_temperature_[K]/1, K to degC/1
  T/1 -> Memory1/1
  [OuterWall_Depth] -> Gain/1
  Ambient_temperature_[K]/1 -> Mux4/3
  [OuterWall_Depth] -> Mux9/1
  Product/1 -> Mux3/2
  [Cp_cement] -> Mux3/3
  "(dT/dt)=Q_sum/{m(Cp)}"/1 -> T/1
  Mux9/1 -> East_wall_volume/1
  [density_cement] -> Product/1
  Mux3/1 -> "(dT/dt)=Q_sum/{m(Cp)}"/1
  East_Out_Convective_coefficient_h/1 -> Mux4/1
  Mux6/1 -> Q_sum=hA(dT)+(k/L)A(dT)+Q_solar =m(Cp)(dT/dt)/1
  [solar_angle_East_to_West] -> Switch/2, Switch1/2
  Switch1/1 -> Switch/1
  Not_shadowed/1 -> Switch1/3
  Shadowed/1 -> Switch/3, Switch1/1
  Switch/1 -> Divide/4
  [Ambient_Temp_K] -> T/2

== system building_HVAC_V00_027_AI_2019b/Building_Block/East_Wall_Block/Subsystem3 ==
  East_Insulator_temperature_[K] : Inport
  Inner_air_temperature_[K] : Inport  Port=2
  East_Inner_Convective_coefficient_h : Inport  Port=3
  "(1/R)=1/{L/(kA)_concrete+L/(kA)_insulator}" : Fcn  Expr=1/(u(1)/u(2)/u(3)+u(4)/u(5)/u(3))
  "(dT/dt)=Q_sum/{m(Cp)}" : Fcn  Expr=u(1)/u(2)/u(3)
  200K to 400K : Saturate  UpperLimit=400  LowerLimit=200
  Divide : Product  Inputs=**
  East_wall_volume : Fcn  Expr=u(1)*u(2)
  Gain : Gain  Gain=0.5
  Gain1 : Gain  Gain=0.5
  K to degC : Fcn  Expr=u(1)-273
  Memory1 : Memory  InitialCondition=300  InheritSampleTime=on
  Mux3 : Mux  Inputs=3
  Mux4 : Mux
  Mux5 : Mux  Inputs=3
  Mux6 : Mux  Inputs=3
  Mux7 : Mux  Inputs=5
  Mux9 : Mux  Inputs=2
  Product : Product
  Q=(1/R)(dT) =(k/L)A(dT) : Fcn  Expr=u(1)*(u(2)-u(3))
  Q=hA(dT) : Fcn  Expr=u(1)*u(2)*(u(3)-u(4))
  Q_sum=hA(dT)+(k/L)A(dT)+Q_solar =m(Cp)(dT/dt) : Fcn  Expr=u(1)+u(2)
  T : Integrator  InitialConditionSource=external
  East_inner_concrete_wall_temperature_[K] : Outport
  East_inner_concrete_wall_temperature_[degC] : Outport  Port=2
  wires:
  Mux6/1 -> Q_sum=hA(dT)+(k/L)A(dT)+Q_solar =m(Cp)(dT/dt)/1
  East_Inner_Convective_coefficient_h/1 -> Mux4/1
  Mux3/1 -> "(dT/dt)=Q_sum/{m(Cp)}"/1
  [density_cement] -> Product/1
  Mux9/1 -> East_wall_volume/1
  "(dT/dt)=Q_sum/{m(Cp)}"/1 -> T/1
  [Cp_cement] -> Mux3/3
  Product/1 -> Mux3/2
  [InnerWall_Depth] -> Mux9/1
  [Area_East] -> Mux4/2, Mux7/3, Mux9/2
  Inner_air_temperature_[K]/1 -> Mux4/3
  [InnerWall_Depth] -> Gain/1
  T/1 -> Memory1/1
  200K to 400K/1 -> K to degC/1, East_inner_concrete_wall_temperature_[K]/1, Mux4/4, Mux5/3
  Mux5/1 -> Q=(1/R)(dT) =(k/L)A(dT)/1
  Mux4/1 -> Q=hA(dT)/1
  Q=(1/R)(dT) =(k/L)A(dT)/1 -> Mux6/2
  Memory1/1 -> 200K to 400K/1
  [Insulator_Depth] -> Gain1/1
  Gain/1 -> Mux7/1
  "(1/R)=1/{L/(kA)_concrete+L/(kA)_insulator}"/1 -> Mux5/1
  Q=hA(dT)/1 -> Mux6/1
  Mux7/1 -> "(1/R)=1/{L/(kA)_concrete+L/(kA)_insulator}"/1
  [k_cement] -> Mux7/2
  Q_sum=hA(dT)+(k/L)A(dT)+Q_solar =m(Cp)(dT/dt)/1 -> Mux3/1
  East_Insulator_temperature_[K]/1 -> Mux5/2
  Gain1/1 -> Mux7/4
  [k_insulator] -> Mux7/5
  East_wall_volume/1 -> Product/2
  K to degC/1 -> East_inner_concrete_wall_temperature_[degC]/1
  [Ambient_Temp_K] -> T/2
  [absorptivity_inner_wall_East] -> Divide/2
  [Q_solar_to_InnerAir] -> Divide/1
  Divide/1 -> Mux6/3

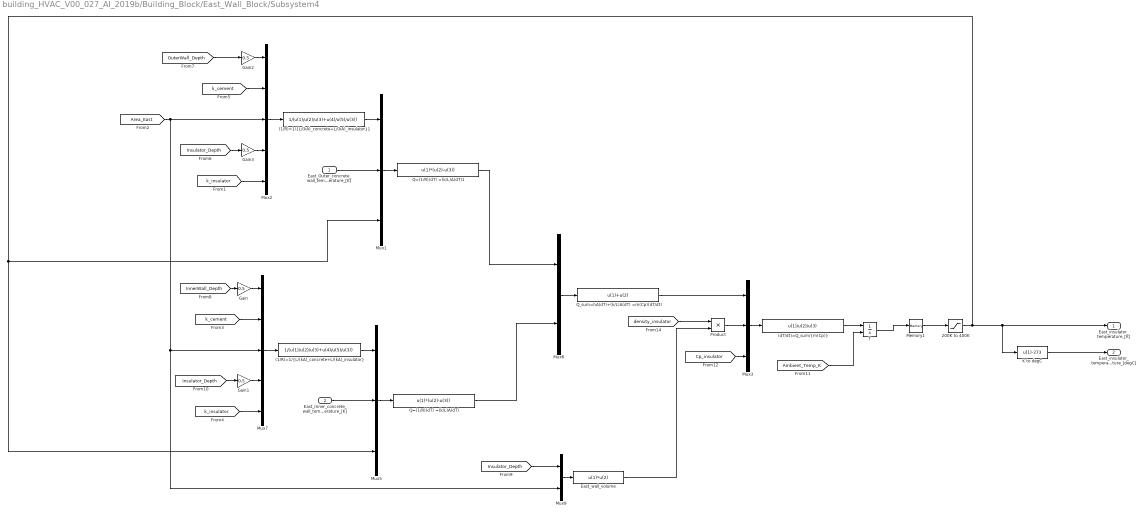
== system building_HVAC_V00_027_AI_2019b/Building_Block/East_Wall_Block/Subsystem4 ==
  East_Outer_concrete_wall_temperature_[K] : Inport
  East_Inner_concrete_wall_temperature_[K] : Inport  Port=2
  "(1/R)=1/{L/(kA)_concrete+L/(kA)_insulator}" : Fcn  Expr=1/(u(1)/u(2)/u(3)+u(4)/u(5)/u(3))
  "(1/R)=1/{L/(kA)_concrete+L/(kA)_insulator}1" : Fcn  Expr=1/(u(1)/u(2)/u(3)+u(4)/u(5)/u(3))
  "(dT/dt)=Q_sum/{m(Cp)}" : Fcn  Expr=u(1)/u(2)/u(3)
  200K to 400K : Saturate  UpperLimit=400  LowerLimit=200
  East_wall_volume : Fcn  Expr=u(1)*u(2)
  Gain{,1..3} (4 alike) : Gain  Gain=0.5
  K to degC : Fcn  Expr=u(1)-273
  Memory1 : Memory  InitialCondition=300  InheritSampleTime=on
  Mux1 : Mux  Inputs=3
  Mux2 : Mux  Inputs=5
  Mux3 : Mux  Inputs=3
  Mux5 : Mux  Inputs=3
  Mux6 : Mux  Inputs=2
  Mux7 : Mux  Inputs=5
  Mux9 : Mux  Inputs=2
  Product : Product
  Q=(1/R)(dT) =(k/L)A(dT) : Fcn  Expr=u(1)*(u(2)-u(3))
  Q=(1/R)(dT) =(k/L)A(dT)1 : Fcn  Expr=u(1)*(u(2)-u(3))
  Q_sum=hA(dT)+(k/L)A(dT) =m(Cp)(dT/dt) : Fcn  Expr=u(1)+u(2)
  T : Integrator  InitialConditionSource=external
  East_insulator_temperature_[K] : Outport
  East_insulator_temperature_[degC] : Outport  Port=2
  wires:
  [OuterWall_Depth] -> Gain2/1
  Gain3/1 -> Mux2/4
  Mux2/1 -> "(1/R)=1/{L/(kA)_concrete+L/(kA)_insulator}1"/1
  East_Outer_concrete_wall_temperature_[K]/1 -> Mux1/2
  Mux1/1 -> Q=(1/R)(dT) =(k/L)A(dT)1/1
  [Insulator_Depth] -> Gain3/1
  [k_cement] -> Mux2/2
  Gain2/1 -> Mux2/1
  "(1/R)=1/{L/(kA)_concrete+L/(kA)_insulator}1"/1 -> Mux1/1
  [k_insulator] -> Mux2/5
  K to degC/1 -> East_insulator_temperature_[degC]/1
  East_wall_volume/1 -> Product/2
  [k_insulator] -> Mux7/5
  Gain1/1 -> Mux7/4
  East_Inner_concrete_wall_temperature_[K]/1 -> Mux5/2
  Q_sum=hA(dT)+(k/L)A(dT) =m(Cp)(dT/dt)/1 -> Mux3/1
  [k_cement] -> Mux7/2
  Mux7/1 -> "(1/R)=1/{L/(kA)_concrete+L/(kA)_insulator}"/1
  Q=(1/R)(dT) =(k/L)A(dT)1/1 -> Mux6/1
  "(1/R)=1/{L/(kA)_concrete+L/(kA)_insulator}"/1 -> Mux5/1
  Gain/1 -> Mux7/1
  [Insulator_Depth] -> Gain1/1
  Memory1/1 -> 200K to 400K/1
  Q=(1/R)(dT) =(k/L)A(dT)/1 -> Mux6/2
  Mux5/1 -> Q=(1/R)(dT) =(k/L)A(dT)/1
  200K to 400K/1 -> Mux5/3, Mux1/3, East_insulator_temperature_[K]/1, K to degC/1
  T/1 -> Memory1/1
  [InnerWall_Depth] -> Gain/1
  [Area_East] -> Mux2/3, Mux7/3, Mux9/2
  [Insulator_Depth] -> Mux9/1
  Product/1 -> Mux3/2
  [Cp_insulator] -> Mux3/3
  "(dT/dt)=Q_sum/{m(Cp)}"/1 -> T/1
  Mux9/1 -> East_wall_volume/1
  [density_insulator] -> Product/1
  Mux3/1 -> "(dT/dt)=Q_sum/{m(Cp)}"/1
  Mux6/1 -> Q_sum=hA(dT)+(k/L)A(dT) =m(Cp)(dT/dt)/1
  [Ambient_Temp_K] -> T/2

== system building_HVAC_V00_027_AI_2019b/Building_Block/Floorl_Block/Subsystem1 ==
  Floor_inner_concrete_wall_temperature_[K] : Inport
  Inner_air_temperature_[K] : Inport  Port=2
  West_Inner_Convective_coefficient_h : Inport  Port=3
  -1000000 to 1000000 : Saturate  UpperLimit=1000000  LowerLimit=-1000000
  Memory : Memory  InheritSampleTime=on
  Mux4 : Mux
  Q=hA(dT) : Fcn  Expr=u(1)*u(2)*(u(3)-u(4))
  Q_Floor_InnerWall_to_InnerAir_[W] : Outport
  wires:
  West_Inner_Convective_coefficient_h/1 -> Mux4/1
  [Area_floor] -> Mux4/2
  Floor_inner_concrete_wall_temperature_[K]/1 -> Mux4/3
  -1000000 to 1000000/1 -> Q_Floor_InnerWall_to_InnerAir_[W]/1
  Mux4/1 -> Q=hA(dT)/1
  Q=hA(dT)/1 -> Memory/1
  Memory/1 -> -1000000 to 1000000/1
  Inner_air_temperature_[K]/1 -> Mux4/4
